simulink model "ContoleLateralApplication_atual"  (R2021a)
settings: Solver=ode23tb  StartTime=0.0  StopTime=TME.Simulation  FixedStep=.001  RelTol=1e-3  EnableMultiTasking=on
StartFcn:
  | %tic
StopFcn:
  | %toc
model workspace (MAT data in the model file):
  A_mu = 10
  B_reff = 8.386
  Cz = 7766.25
  DCT_Param : object (value not decoded)
  DLCXref = [0 6 7 14 33.5 34 42 50 60]
  DLCYref = [0 0 -4.5 -4 -3.75 1.5 0.5 0 0]
  D_reff = 0.25826
  Downshift_Speeds = [9.5625 12.9375 16.3125 19.6875 23.0625 26.4375 29.8125 33.1875 36.5625 39.9375 43.3125 46.6875 ... (28 elements, 4x7)]
  EngRevLim = 7000
  Pedal_Positions = [0.1 0.4 0.5 0.9]
  SUS : object (value not decoded)
  Upshift_Speeds = [12.9375 16.3125 19.6875 33 26.4375 29.8125 33.1875 52.5 39.9375 43.3125 46.6875 77.25 ... (28 elements, 4x7)]
  VEH : object (value not decoded)
  V_o = 16.7
  V_xlow = 1
  WH : object (value not decoded)
  a = 1.4
  alpha_max = 1.5
  alpha_min = -1.5
  b = 1.8
  c_zo = 209651
  epsilon = 0.1
  h = 0.134
  path : object (value not decoded)
  pio = 220000
  q_Fcx = 0
  q_Fz2 = 15.4
  q_Fzy = 0
  q_reo = 0.9974
  q_sx1 = -0.007764
  q_sx10 = 0.2824
  q_sx11 = 5.349
  q_sx12 = 0
  q_sx13 = 0
  q_sx14 = 0
  q_sx2 = 1.1915
  q_sx3 = 0.013948
  q_sx4 = 4.912
  q_sx5 = 1.02
  q_sx6 = 22.83
  q_sx7 = 0.7104
  q_sx8 = -0.023393
  q_sx9 = 0.6581
  q_sy1 = 0.00702
  q_sy2 = 0
  q_sy3 = 0.001515
  q_sy4 = 8.514e-05
  q_sy5 = 0
  q_sy6 = 0
  q_sy7 = 0.9008
  q_sy8 = -0.4089
  q_v1 = 0.0007742
  q_v2 = 0.04667
  r_Bx1 = 12.531
  r_Bx2 = 9.532
  r_Bx3 = 0
  r_By1 = 10.615
  r_By2 = 7.705
  r_By3 = 3.433e-06
  r_By4 = 0
  r_Cx1 = 1.019
  r_Cy1 = 1.0585
  r_Ex1 = -0.4487
  r_Ex2 = -0.4726
  r_Ey1 = 0.3132
  r_Ey2 = 7.63e-06
  r_Hx1 = 0.0002374
  r_Hy1 = 0.011646
  r_Hy2 = 7.63e-06
  r_Vy1 = 0.05654
  r_Vy2 = 7.63e-06
  r_Vy3 = 0
  r_Vy4 = 99.9
  r_Vy5 = 2
  r_Vy6 = 15.814
  r_o = 0.3135
  vehWidth = 2
  w = 1
values from neighbouring files (symbols this model uses):
  C1 = 1.2801    [Data_ControleLateral_atual.m]
  C2 = 23.99    [Data_ControleLateral_atual.m]
  C3 = 0.52    [Data_ControleLateral_atual.m]
symbols that are objects in the model workspace (value not decoded): VEH
undefined symbols (not defined in the file or in its folder): Disabled, EV, GND, MTR, Right, SENSOR, STEER, WHL
libraries: autolibutils x5, vehdynlibscenariocommon x5, autolibshared x5, sim3dlib x4, vehdynlibtirecommon x2, autolibmappedmotor x2, vehdynlibviscommon x2, vehdynlibsteering x1, pid_lib x1, vehdynlibdriver x1, vehdynlibsens x1, sharedtransform x1
(part 5 of 6)

== system ContoleLateralApplication_atual/Veh2Tire ==
  Axle : Inport
  r : Inport  Port=2
  VehVel : Inport  Port=3
  WheelSteer : Inport  Port=4
  Reshape4 : Reshape
  Unary Minus : UnaryMinus
  Wheel to Body Transform : Subsystem
  T : Outport  VectorParamsAs1DForOutWhenUnconnected=off
  xdotAxle : Outport  Port=2  VectorParamsAs1DForOutWhenUnconnected=off
  ydotAxle : Outport  Port=3  VectorParamsAs1DForOutWhenUnconnected=off
  psidot : Outport  Port=4  VectorParamsAs1DForOutWhenUnconnected=off
  zdotAxle : Outport  Port=5  VectorParamsAs1DForOutWhenUnconnected=off
  wires:
  Axle/1 -> Reshape4/1
  Wheel to Body Transform/1(xdotWheel) -> xdotAxle/1  "Vx"
  Wheel to Body Transform/2(ydotWheel) -> ydotAxle/1  "Vy"
  r/1 -> Unary Minus/1
  Reshape4/1 -> T/1
  VehVel/1 -> Wheel to Body Transform/1(VelVeh)
  WheelSteer/1 -> Wheel to Body Transform/2(WheelAngles)
  Wheel to Body Transform/3(zdotWheel) -> zdotAxle/1  "Vz"
  Unary Minus/1 -> psidot/1

== system ContoleLateralApplication_atual/Velocity and Vertical Load ==
  note: 1) Add Subsystem or Model blocks as valid variant choices.
      | 2) You cannot connect blocks at this level. At simulation, connectivity is automatically
      | determined, based on the active variant and port name matching.
  VehFdbk : Inport
  Bicycle : Subsystem  VariantControl=0
  Dual : Subsystem  VariantControl=1
  VehV : Outport  VectorParamsAs1DForOutWhenUnconnected=off
  Fz : Outport  Port=2  PortDimensions=4  VectorParamsAs1DForOutWhenUnconnected=off

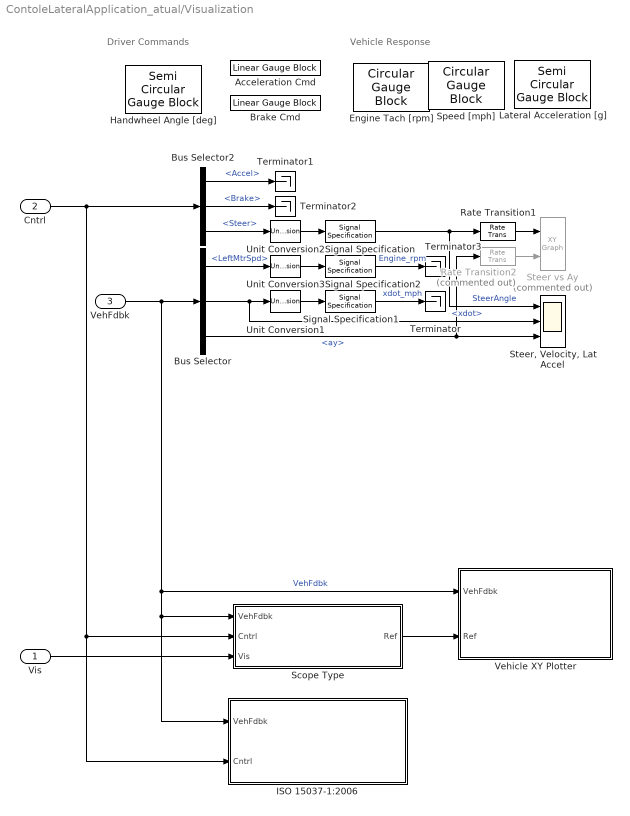
== system ContoleLateralApplication_atual/Visualization ==
  note: Vehicle Response
  note: Driver Commands
  Vis : Inport
  Cntrl : Inport  Port=2
  VehFdbk : Inport  Port=3
  Acceleration Cmd : LinearGaugeBlock  LabelPosition=Hide  ScaleMax=1  TickInterval=0.20000000000000001
  Brake Cmd : LinearGaugeBlock  LabelPosition=Hide  ScaleMax=1  TickInterval=0.20000000000000001
  Bus Selector : BusSelector  OutputSignals=Driveline.LeftMtrSpd,Chassis.xdot,Chassis.ay
  Bus Selector2 : BusSelector  OutputSignals=Accel,Brake,Steer
  Engine Tach [rpm] : CircularGaugeBlock  LabelPosition=Hide  ScaleMax=8000  TickInterval=1000
  Handwheel Angle [deg] : SemiCircularGaugeBlock  LabelPosition=Hide  ScaleMin=-300  ScaleMax=300  TickInterval=60
  ISO 15037-1:2006 : Subsystem  StopFcn=|  Variant=on  VariantControlMode=label  LabelModeActiveChoice=0  mask(ISO 15037-1:2006){Measurement=Disabled}
      | switch get_param(gcb,'Measurement')
      |     case 'Enabled'
      |        p=slproject.getCurrentProject;
      |        projectRoot=p.RootFolder;
      |        SySFolder=fullfile(projectRoot, 'System');
      |        Simulink.sdi.loadView([SySFolder filesep 'ISO15037_1_2006E.mldatx']);
      |        Simulink.sdi.view;
      | end
      mask prompts: Measurement "ISO Measurements"
      mask help: Enables display of ISO 15037-1:2006 standard measurement signals in the Simulation Data Inspector.
      mask init:
      | switch get_param(gcb,'Measurement')
      |     case 'Disabled'
      |         set_param(gcb,'OverrideUsingVariant','0')
      |     case 'Enabled'
      |        set_param(gcb,'OverrideUsingVariant','1')
      |     otherwise
      |        set_param(gcb,'OverrideUsingVariant','0')
      | end
      settings: AttributesFormatString=%<Measurement>
      mask Help: eval('vdynblkshelp(''iso15037'')');
      mask TypeOptions Measurement: Enabled | Disabled
      mask Callback Measurement:
      | switch get_param(gcb,'Measurement')
      |     case 'Disabled'
      |         set_param(gcb,'OverrideUsingVariant','0')
      |     case 'Enabled'
      |        set_param(gcb,'OverrideUsingVariant','1')
      |     otherwise
      |        set_param(gcb,'OverrideUsingVariant','0')
      | end
      mask Display: disp('ISO 15037-1:2006')
  Lateral Acceleration [g] : SemiCircularGaugeBlock  LabelPosition=Hide  ScaleMin=-1  ScaleMax=1  TickInterval=0.5
  Rate Transition1 : RateTransition  Deterministic=off  OutPortSampleTime=.1
  Rate Transition2 : RateTransition  Commented=on  Deterministic=off  OutPortSampleTime=.1
  Scope Type : Subsystem  Variant=on  VariantControlMode=label  VariantControl=Variant1  LabelModeActiveChoice=2
  Signal Specification : SignalSpecification  Unit=deg
  Signal Specification1 : SignalSpecification  Unit=mph
  Signal Specification2 : SignalSpecification  Unit=rpm
  Speed [mph] : CircularGaugeBlock  LabelPosition=Hide  TickInterval=10
  Steer vs Ay : simulink/Sinks/XY Graph  Commented=on  xmin=-300  xmax=300  ymin=-1.5  ymax=1.5  st=.1
  "Steer, Velocity, Lat Accel" : Scope  NumInputPorts=3
  Terminator{,1..3} (4 alike) : Terminator
  Unit Conversion1 : UnitConversion
  Unit Conversion2 : UnitConversion
  Unit Conversion3 : UnitConversion
  Vehicle XY Plotter : Subsystem  Variant=on  VariantControlMode=label  VariantControl=Variant1  LabelModeActiveChoice=1
  wires:
  Signal Specification/1 -> Rate Transition1/1, "Steer, Velocity, Lat Accel"/1  "SteerAngle"
  Bus Selector/3 -> Rate Transition2/1, "Steer, Velocity, Lat Accel"/3  "<ay>"
  Bus Selector/2 -> "Steer, Velocity, Lat Accel"/2, Unit Conversion1/1  "<xdot>"
  Unit Conversion2/1 -> Signal Specification/1
  Unit Conversion1/1 -> Signal Specification1/1
  Signal Specification1/1 -> Terminator/1  "xdot_mph"
  Bus Selector2/3 -> Unit Conversion2/1  "<Steer>"
  Rate Transition1/1 -> Steer vs Ay/1
  Rate Transition2/1 -> Steer vs Ay/2
  Bus Selector2/1 -> Terminator1/1  "<Accel>"
  Bus Selector2/2 -> Terminator2/1  "<Brake>"
  Signal Specification2/1 -> Terminator3/1  "Engine_rpm"
  Unit Conversion3/1 -> Signal Specification2/1
  Bus Selector/1 -> Unit Conversion3/1  "<LeftMtrSpd>"
  VehFdbk/1 -> ISO 15037-1:2006/1(VehFdbk), Scope Type/1("VehFdbk "), Vehicle XY Plotter/1("VehFdbk "), Bus Selector/1  "VehFdbk"
  Cntrl/1 -> ISO 15037-1:2006/2(Cntrl), Scope Type/2(Cntrl), Bus Selector2/1
  Vis/1 -> Scope Type/3("Vis ")
  Scope Type/1(" Ref") -> Vehicle XY Plotter/2("Ref ")

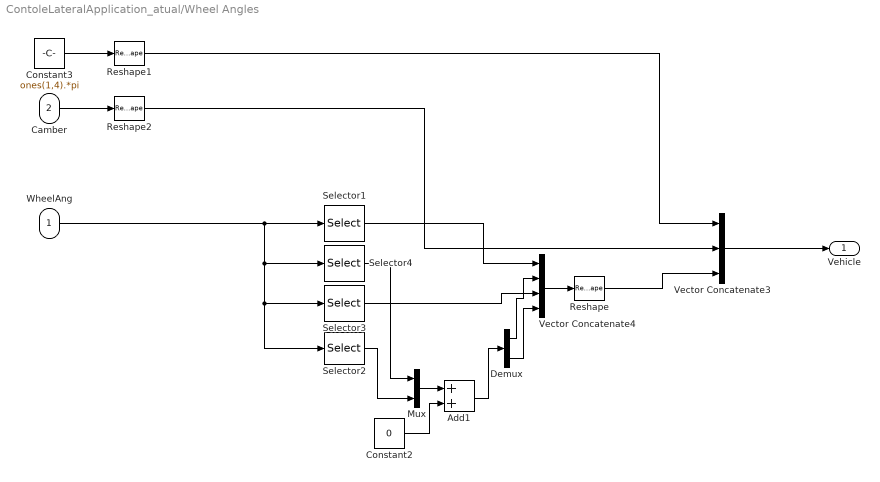
== system ContoleLateralApplication_atual/Wheel Angles ==
  WheelAng : Inport
  Camber : Inport  Port=2
  Add1 : Sum
  Constant2 : Constant  Value=0
  Constant3 : Constant  Value=ones(1,4).*pi
  Demux : Demux  Outputs=2
  Mux : Mux  Inputs=2
  Reshape : Reshape  OutputDimensionality=Row vector (2-D)
  Reshape1 : Reshape  OutputDimensionality=Row vector (2-D)
  Reshape2 : Reshape  OutputDimensionality=Row vector (2-D)
  Selector1 : Selector  InputPortWidth=4  IndexOptions=Index vector (dialog)  Indices=1  OutputSizes=4
  Selector2 : Selector  InputPortWidth=4  IndexOptions=Index vector (dialog)  Indices=4  OutputSizes=4
  Selector3 : Selector  InputPortWidth=4  IndexOptions=Index vector (dialog)  Indices=3  OutputSizes=4
  Selector4 : Selector  InputPortWidth=4  IndexOptions=Index vector (dialog)  Indices=2  OutputSizes=4
  Vector Concatenate3 : Concatenate  NumInputs=3  Mode=Multidimensional array
  Vector Concatenate4 : Concatenate  NumInputs=4
  Vehicle : Outport  VectorParamsAs1DForOutWhenUnconnected=off
  wires:
  Selector4/1 -> Mux/1
  Constant2/1 -> Add1/2
  Add1/1 -> Demux/1
  Selector3/1 -> Vector Concatenate4/3
  Selector1/1 -> Vector Concatenate4/1
  Mux/1 -> Add1/1
  Selector2/1 -> Mux/2
  Demux/1 -> Vector Concatenate4/2
  Demux/2 -> Vector Concatenate4/4
  Vector Concatenate4/1 -> Reshape/1
  Constant3/1 -> Reshape1/1
  Vector Concatenate3/1 -> Vehicle/1
  Reshape/1 -> Vector Concatenate3/3
  Reshape1/1 -> Vector Concatenate3/1
  Reshape2/1 -> Vector Concatenate3/2
  Camber/1 -> Reshape2/1
  WheelAng/1 -> Selector2/1, Selector3/1, Selector4/1, Selector1/1

== system ContoleLateralApplication_atual/Wheel Positions ==
  Info : Inport
  Bus Selector : BusSelector  OutputSignals=InertFrm.FrntAxl.Lft.Disp.Y,InertFrm.FrntAxl.Rght.Disp.Y,InertFrm.RearAxl.Lft.Disp.Y,InertFrm.RearAxl.Rght.Disp.Y
  Bus Selector1 : BusSelector  OutputSignals=InertFrm.FrntAxl.Lft.Disp.X,InertFrm.FrntAxl.Rght.Disp.X,InertFrm.RearAxl.Lft.Disp.X,InertFrm.RearAxl.Rght.Disp.X
  Vector Concatenate1 : Concatenate  NumInputs=4
  Vector Concatenate2 : Concatenate  NumInputs=4
  XWheel : Outport  Unit=m  VectorParamsAs1DForOutWhenUnconnected=off
  YWheel : Outport  Port=2  Unit=m  VectorParamsAs1DForOutWhenUnconnected=off
  wires:
  Bus Selector1/4 -> Vector Concatenate2/4  "<X>"
  Bus Selector/1 -> Vector Concatenate1/1  "<Y>"
  Bus Selector1/3 -> Vector Concatenate2/3  "<X>"
  Bus Selector/4 -> Vector Concatenate1/4  "<Y>"
  Bus Selector1/2 -> Vector Concatenate2/2  "<X>"
  Bus Selector/3 -> Vector Concatenate1/3  "<Y>"
  Bus Selector/2 -> Vector Concatenate1/2  "<Y>"
  Vector Concatenate1/1 -> YWheel/1
  Info/1 -> Bus Selector/1, Bus Selector1/1
  Bus Selector1/1 -> Vector Concatenate2/1  "<X>"
  Vector Concatenate2/1 -> XWheel/1

== system ContoleLateralApplication_atual/Axle Forces/Bicycle ==
  F : Inport
  R : Inport  Port=2
  Sum of Elements : Sum  Inputs=+
  Sum of Elements1 : Sum  Inputs=+
  FrntAxlF : Outport  Unit=N  VectorParamsAs1DForOutWhenUnconnected=off
  RearAxlF : Outport  Port=2  Unit=N  VectorParamsAs1DForOutWhenUnconnected=off
  wires:
  Sum of Elements/1 -> FrntAxlF/1
  Sum of Elements1/1 -> RearAxlF/1
  R/1 -> Sum of Elements1/1
  F/1 -> Sum of Elements/1

== system ContoleLateralApplication_atual/Axle Forces/Dual ==
  F : Inport
  R : Inport  Port=2
  FrntAxlF : Outport  Unit=N  VectorParamsAs1DForOutWhenUnconnected=off
  RearAxlF : Outport  Port=2  Unit=N  VectorParamsAs1DForOutWhenUnconnected=off
  wires:
  R/1 -> RearAxlF/1
  F/1 -> FrntAxlF/1

== system ContoleLateralApplication_atual/Environment/Ground Feedback ==
  note: 1) Add Subsystem or Model blocks as valid variant choices.
      | 2) You cannot connect blocks at this level. At simulation, connectivity is automatically
      | determined, based on the active variant and port name matching.
  Friction : Inport
  3D Engine : Subsystem  VariantControl=1
  Constant : Subsystem  VariantControl=0
  Ground : Outport  VectorParamsAs1DForOutWhenUnconnected=off

== system ContoleLateralApplication_atual/Reference Generator/3D Engine ==
  note: 1) Add Subsystem or Model blocks as valid variant choices.
      | 2) You cannot connect blocks at this level. At simulation, connectivity is automatically
      | determined, based on the active variant and port name matching.
  VehFdbk : Inport
  3D Engine : Subsystem  VariantControl=1
  3D Engine Disabled : Subsystem  VariantControl=0

== system ContoleLateralApplication_atual/Reference Generator/Reference Generator ==
  "VehFdbk " : Inport
  Constant Radius : vehdynlibscenariocommon/Constant Radius  VariantControl=4  t_start=t_start  xdot_r=xdot_r  xdotUnit=mph  R=R  turnDirMask=Right  ay_max=cr_ay_max  ay_stop=off  Parameter6=2
      settings: SourceProductBaseCode=VE
  Double Lane Change : Subsystem  VariantControl=0
  Increasing Steer : Subsystem  VariantControl=1
  Sine with Dwell : Subsystem  VariantControl=3
  Swept Sine : Subsystem  VariantControl=2
  " Vis" : Outport  VectorParamsAs1DForOutWhenUnconnected=off
  " Ref" : Outport  Port=2  VectorParamsAs1DForOutWhenUnconnected=off
  " Fdbk" : Outport  Port=3  VectorParamsAs1DForOutWhenUnconnected=off

== system ContoleLateralApplication_atual/Tires/Fx ==
  In1 : Inport
  In2 : Inport  Port=2
  In3 : Inport  Port=3
  In4 : Inport  Port=4
  Bus Selector{,1..3} (4 alike) : BusSelector  OutputSignals=Fx
  Vector Concatenate : Concatenate  NumInputs=4
  Out1 : Outport  VectorParamsAs1DForOutWhenUnconnected=off
  wires:
  Bus Selector3/1 -> Vector Concatenate/4  "<Fx>"
  Bus Selector2/1 -> Vector Concatenate/3  "<Fx>"
  Bus Selector1/1 -> Vector Concatenate/2  "<Fx>"
  In4/1 -> Bus Selector3/1
  In3/1 -> Bus Selector2/1
  In2/1 -> Bus Selector1/1
  Bus Selector/1 -> Vector Concatenate/1  "<Fx>"
  In1/1 -> Bus Selector/1
  Vector Concatenate/1 -> Out1/1

== system ContoleLateralApplication_atual/Tires/Fz1 ==
  In1 : Inport
  In2 : Inport  Port=2
  In3 : Inport  Port=3
  In4 : Inport  Port=4
  Bus Selector{,1..3} (4 alike) : BusSelector  OutputSignals=Fz
  Vector Concatenate : Concatenate  NumInputs=4
  Out1 : Outport  VectorParamsAs1DForOutWhenUnconnected=off
  wires:
  Vector Concatenate/1 -> Out1/1
  In1/1 -> Bus Selector/1
  Bus Selector/1 -> Vector Concatenate/1  "<Fz>"
  In2/1 -> Bus Selector1/1
  In3/1 -> Bus Selector2/1
  In4/1 -> Bus Selector3/1
  Bus Selector1/1 -> Vector Concatenate/2  "<Fz>"
  Bus Selector2/1 -> Vector Concatenate/3  "<Fz>"
  Bus Selector3/1 -> Vector Concatenate/4  "<Fz>"

== system ContoleLateralApplication_atual/Tires/My ==
  In1 : Inport
  In2 : Inport  Port=2
  In3 : Inport  Port=3
  In4 : Inport  Port=4
  Bus Selector{,1..3} (4 alike) : BusSelector  OutputSignals=My
  Vector Concatenate : Concatenate  NumInputs=4
  Out1 : Outport  PortDimensions=4  VectorParamsAs1DForOutWhenUnconnected=off
  wires:
  Bus Selector3/1 -> Vector Concatenate/4  "<My>"
  Bus Selector2/1 -> Vector Concatenate/3  "<My>"
  Bus Selector1/1 -> Vector Concatenate/2  "<My>"
  In4/1 -> Bus Selector3/1
  In3/1 -> Bus Selector2/1
  In2/1 -> Bus Selector1/1
  Bus Selector/1 -> Vector Concatenate/1  "<My>"
  In1/1 -> Bus Selector/1
  Vector Concatenate/1 -> Out1/1

== system ContoleLateralApplication_atual/Tires/Re ==
  In1 : Inport
  In2 : Inport  Port=2
  In3 : Inport  Port=3
  In4 : Inport  Port=4
  Bus Selector{,1..3} (4 alike) : BusSelector  OutputSignals=Re
  Vector Concatenate : Concatenate  NumInputs=4
  Out1 : Outport  PortDimensions=4  VectorParamsAs1DForOutWhenUnconnected=off
  wires:
  Vector Concatenate/1 -> Out1/1
  In1/1 -> Bus Selector/1
  Bus Selector/1 -> Vector Concatenate/1  "<Re>"
  In2/1 -> Bus Selector1/1
  In3/1 -> Bus Selector2/1
  In4/1 -> Bus Selector3/1
  Bus Selector1/1 -> Vector Concatenate/2  "<Re>"
  Bus Selector2/1 -> Vector Concatenate/3  "<Re>"
  Bus Selector3/1 -> Vector Concatenate/4  "<Re>"

== system ContoleLateralApplication_atual/Tires/alpha ==
  In1 : Inport
  In2 : Inport  Port=2
  In3 : Inport  Port=3
  In4 : Inport  Port=4
  Vector Concatenate : Concatenate  NumInputs=4
  Out1 : Outport  PortDimensions=4  VectorParamsAs1DForOutWhenUnconnected=off
  wires:
  Vector Concatenate/1 -> Out1/1
  In1/1 -> Vector Concatenate/1
  In2/1 -> Vector Concatenate/2
  In3/1 -> Vector Concatenate/3
  In4/1 -> Vector Concatenate/4

== system ContoleLateralApplication_atual/Tires/kappa ==
  In1 : Inport
  In2 : Inport  Port=2
  In3 : Inport  Port=3
  In4 : Inport  Port=4
  Bus Selector{,1..3} (4 alike) : BusSelector  OutputSignals=Kappa
  Vector Concatenate : Concatenate  NumInputs=4
  Out1 : Outport  PortDimensions=4  VectorParamsAs1DForOutWhenUnconnected=off
  wires:
  Bus Selector3/1 -> Vector Concatenate/4  "<Kappa>"
  Bus Selector2/1 -> Vector Concatenate/3  "<Kappa>"
  Bus Selector1/1 -> Vector Concatenate/2  "<Kappa>"
  In4/1 -> Bus Selector3/1
  In3/1 -> Bus Selector2/1
  In2/1 -> Bus Selector1/1
  Bus Selector/1 -> Vector Concatenate/1  "<Kappa>"
  In1/1 -> Bus Selector/1
  Vector Concatenate/1 -> Out1/1

== system ContoleLateralApplication_atual/Tires/omega ==
  In1 : Inport
  In2 : Inport  Port=2
  In3 : Inport  Port=3
  In4 : Inport  Port=4
  Bus Selector{1..4} (4 alike) : BusSelector  OutputSignals=Omega
  Vector Concatenate : Concatenate  NumInputs=4
  Out1 : Outport  VectorParamsAs1DForOutWhenUnconnected=off
  wires:
  In1/1 -> Bus Selector4/1
  Bus Selector4/1 -> Vector Concatenate/1  "<Omega>"
  In2/1 -> Bus Selector2/1
  In3/1 -> Bus Selector1/1
  In4/1 -> Bus Selector3/1
  Bus Selector2/1 -> Vector Concatenate/2  "<Omega>"
  Vector Concatenate/1 -> Out1/1
  Bus Selector3/1 -> Vector Concatenate/4  "<Omega>"
  Bus Selector1/1 -> Vector Concatenate/3  "<Omega>"

== system ContoleLateralApplication_atual/Tires/z ==
  In1 : Inport
  In2 : Inport  Port=2
  In3 : Inport  Port=3
  In4 : Inport  Port=4
  Bus Selector{,1..3} (4 alike) : BusSelector  OutputSignals=z
  Vector Concatenate : Concatenate  NumInputs=4
  Out1 : Outport  PortDimensions=4  VectorParamsAs1DForOutWhenUnconnected=off
  wires:
  Bus Selector3/1 -> Vector Concatenate/4  "<z>"
  Bus Selector2/1 -> Vector Concatenate/3  "<z>"
  Bus Selector1/1 -> Vector Concatenate/2  "<z>"
  In4/1 -> Bus Selector3/1
  In3/1 -> Bus Selector2/1
  In2/1 -> Bus Selector1/1
  Bus Selector/1 -> Vector Concatenate/1  "<z>"
  In1/1 -> Bus Selector/1
  Vector Concatenate/1 -> Out1/1

== system ContoleLateralApplication_atual/Tires/zdot ==
  In1 : Inport
  In2 : Inport  Port=2
  In3 : Inport  Port=3
  In4 : Inport  Port=4
  Bus Selector{,1..3} (4 alike) : BusSelector  OutputSignals=zdot
  Vector Concatenate : Concatenate  NumInputs=4
  Out1 : Outport  PortDimensions=4  VectorParamsAs1DForOutWhenUnconnected=off
  wires:
  Vector Concatenate/1 -> Out1/1
  In1/1 -> Bus Selector/1
  Bus Selector/1 -> Vector Concatenate/1  "<zdot>"
  In2/1 -> Bus Selector1/1
  In3/1 -> Bus Selector2/1
  In4/1 -> Bus Selector3/1
  Bus Selector1/1 -> Vector Concatenate/2  "<zdot>"
  Bus Selector2/1 -> Vector Concatenate/3  "<zdot>"
  Bus Selector3/1 -> Vector Concatenate/4  "<zdot>"

== system ContoleLateralApplication_atual/Veh2Tire/Wheel to Body Transform ==
  VelVeh : Inport  Partition=on  PartitionDimension=2  PartitionWidth=1  PartitionOffset=0
  WheelAngles : Inport  Port=2  Partition=on  PartitionDimension=2  PartitionWidth=1  PartitionOffset=0
  Demux1 : Demux  Outputs=3
  Divide1 : Product  Inputs=**  Multiplication=Matrix(*)
  For Each : ForEach  DisableCoverage=on
  Rotation Angles to Direction Cosine Matrix : sharedtransform/Rotation Angles to Direction Cosine Matrix  rotationOrder=ZYX  aMode=2
      settings: SourceProductBaseCode=AE,PW,DR,MT,UV,VE
  Selector : Selector  InputPortWidth=3  IndexOptions=Index vector (dialog)  Indices=[3 2 1]  OutputSizes=1
  xdotWheel : Outport  ConcatenationDimension=1  VectorParamsAs1DForOutWhenUnconnected=off
  ydotWheel : Outport  Port=2  ConcatenationDimension=1  VectorParamsAs1DForOutWhenUnconnected=off
  zdotWheel : Outport  Port=3  ConcatenationDimension=1  VectorParamsAs1DForOutWhenUnconnected=off
  wires:
  Divide1/1 -> Demux1/1
  Demux1/1 -> xdotWheel/1
  Demux1/2 -> ydotWheel/1
  Demux1/3 -> zdotWheel/1
  Rotation Angles to Direction Cosine Matrix/1 -> Divide1/1
  VelVeh/1 -> Divide1/2
  WheelAngles/1 -> Selector/1
  Selector/1 -> Rotation Angles to Direction Cosine Matrix/1

== system ContoleLateralApplication_atual/Velocity and Vertical Load/Bicycle ==
  VehFdbk : Inport
  Bicycle Fz : Subsystem
  Bicycle V : Subsystem
  VehV : Outport  VectorParamsAs1DForOutWhenUnconnected=off
  Fz : Outport  Port=2  VectorParamsAs1DForOutWhenUnconnected=off
  wires:
  Bicycle V/1(Out1) -> VehV/1
  Bicycle Fz/1(Out1) -> Fz/1
  VehFdbk/1 -> Bicycle Fz/1(In1), Bicycle V/1(In1)

== system ContoleLateralApplication_atual/Velocity and Vertical Load/Dual ==
  VehFdbk : Inport
  Dual Fz : Subsystem
  Dual V : Subsystem
  VehV : Outport  VectorParamsAs1DForOutWhenUnconnected=off
  Fz : Outport  Port=2  VectorParamsAs1DForOutWhenUnconnected=off
  wires:
  Dual V/1(Out1) -> VehV/1
  VehFdbk/1 -> Dual Fz/1(In1), Dual V/1(In1)
  Dual Fz/1(Out1) -> Fz/1

== system ContoleLateralApplication_atual/Visualization/ISO 15037-1:2006 ==
  VehFdbk : Inport
  Cntrl : Inport  Port=2
  Disabled : Subsystem  VariantControl=0
  Enabled : Subsystem  VariantControl=1

== system ContoleLateralApplication_atual/Visualization/Scope Type ==
  "VehFdbk " : Inport
  Cntrl : Inport  Port=2
  "Vis " : Inport  Port=3
  DLC : Subsystem  VariantControl=1
  None : Subsystem  VariantControl=0
  XYZ : Subsystem  VariantControl=2
  " Ref" : Outport  VectorParamsAs1DForOutWhenUnconnected=off

== system ContoleLateralApplication_atual/Visualization/Vehicle XY Plotter ==
  "VehFdbk " : Inport
  "Ref " : Inport  Port=2
  XY View : Subsystem  VariantControl=0
  XY View Ref : Subsystem  VariantControl=1

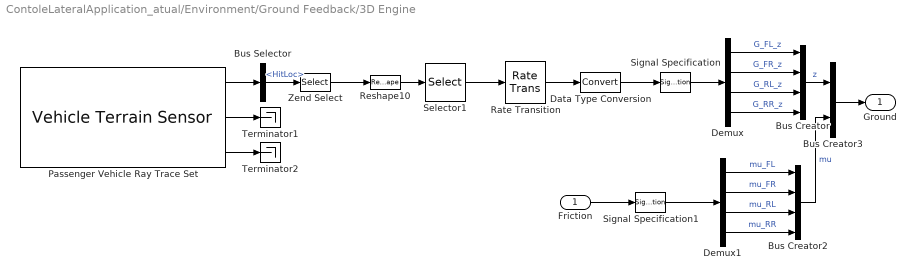
== system ContoleLateralApplication_atual/Environment/Ground Feedback/3D Engine ==
  Friction : Inport
  Bus Creator : BusCreator  Inputs=4
  Bus Creator2 : BusCreator  Inputs=4
  Bus Creator3 : BusCreator  Inputs=2
  Bus Selector : BusSelector  OutputSignals=HitLoc
  Data Type Conversion : DataTypeConversion
  Demux : Demux
  Demux1 : Demux
  Passenger Vehicle Ray Trace Set : sim3dlib/Vehicle Terrain Sensor  ActorTag=SimulinkVehicle1  VehExtEn=Constant  TireRadiiExt=Constant  VehCntrLngthVal=0  TireRadiiVal=0  VehRayLngth=10  LfRayLngth=20  RfRayLngth=20  LrRayLngth=20  RrRayLngth=20  VehRayOffset=0  LfRayOffset=-1  RfRayOffset=-1  LrRayOffset=-1  RrRayOffset=-1  VehEn=on  LfEn=on  RfEn=on  LrEn=on  RrEn=on  DbgEn=off  Ts=.03  aMode=aMode
      settings: SourceProductBaseCode=DR,UV,VE
  Rate Transition : RateTransition
  Reshape10 : Reshape  OutputDimensionality=Row vector (2-D)
  Selector1 : Selector  InputPortWidth=5  IndexOptions=Index vector (dialog)  Indices=[2:5]  OutputSizes=1
  Signal Specification : SignalSpecification  Unit=m
  Signal Specification1 : SignalSpecification  Unit=1
  Terminator1 : Terminator
  Terminator2 : Terminator
  Zend Select : Selector  NumberOfDimensions=2  InputPortWidth=3  IndexOptions=Select all,Index vector (dialog)  Indices=[1 3],3  OutputSizes=1,1
  Ground : Outport  VectorParamsAs1DForOutWhenUnconnected=off
  wires:
  Selector1/1 -> Rate Transition/1
  Zend Select/1 -> Reshape10/1
  Bus Selector/1 -> Zend Select/1  "<HitLoc>"
  Passenger Vehicle Ray Trace Set/2 -> Terminator1/1
  Passenger Vehicle Ray Trace Set/3 -> Terminator2/1
  Reshape10/1 -> Selector1/1
  Passenger Vehicle Ray Trace Set/1 -> Bus Selector/1
  Rate Transition/1 -> Data Type Conversion/1
  Demux/2 -> Bus Creator/2  "G_FR_z"
  Demux/1 -> Bus Creator/1  "G_FL_z"
  Demux/4 -> Bus Creator/4  "G_RR_z"
  Demux/3 -> Bus Creator/3  "G_RL_z"
  Signal Specification/1 -> Demux/1
  Signal Specification1/1 -> Demux1/1
  Demux1/1 -> Bus Creator2/1  "mu_FL"
  Bus Creator/1 -> Bus Creator3/1  "z"
  Demux1/3 -> Bus Creator2/3  "mu_RL"
  Demux1/4 -> Bus Creator2/4  "mu_RR"
  Demux1/2 -> Bus Creator2/2  "mu_FR"
  Bus Creator2/1 -> Bus Creator3/2  "mu"
  Bus Creator3/1 -> Ground/1
  Friction/1 -> Signal Specification1/1
  Data Type Conversion/1 -> Signal Specification/1

== system ContoleLateralApplication_atual/Environment/Ground Feedback/Constant ==
  Friction : Inport
  Bus Creator : BusCreator  Inputs=4
  Bus Creator2 : BusCreator  Inputs=4
  Bus Creator3 : BusCreator  Inputs=2
  Constant1 : Constant  Value=zeros(4,1)
  Demux : Demux
  Demux1 : Demux
  Signal Specification : SignalSpecification  Unit=m
  Signal Specification1 : SignalSpecification  Unit=1
  Ground : Outport  VectorParamsAs1DForOutWhenUnconnected=off
  wires:
  Constant1/1 -> Signal Specification/1
  Signal Specification/1 -> Demux/1
  Demux/4 -> Bus Creator/4  "G_RR_z"
  Demux/1 -> Bus Creator/1  "G_FL_z"
  Demux/3 -> Bus Creator/3  "G_RL_z"
  Demux/2 -> Bus Creator/2  "G_FR_z"
  Bus Creator/1 -> Bus Creator3/1  "z"
  Demux1/3 -> Bus Creator2/3  "mu_RL"
  Demux1/4 -> Bus Creator2/4  "mu_RR"
  Demux1/1 -> Bus Creator2/1  "mu_FL"
  Demux1/2 -> Bus Creator2/2  "mu_FR"
  Bus Creator2/1 -> Bus Creator3/2  "mu"
  Friction/1 -> Signal Specification1/1
  Signal Specification1/1 -> Demux1/1
  Bus Creator3/1 -> Ground/1

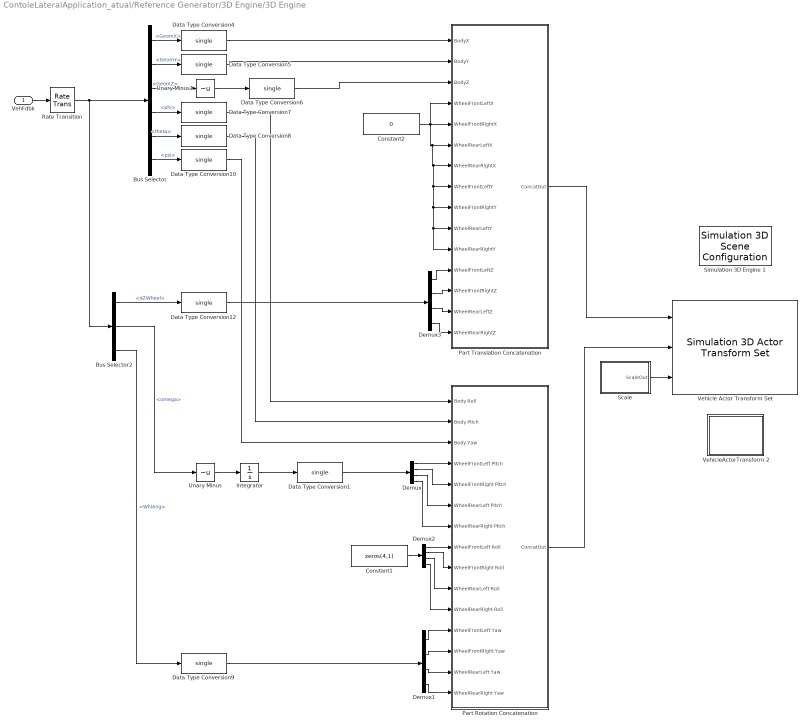
== system ContoleLateralApplication_atual/Reference Generator/3D Engine/3D Engine ==
  VehFdbk : Inport
  Bus Selector : BusSelector  OutputSignals=Body.GeomX,Body.GeomY,Body.GeomZ,Body.phi,Body.theta,Body.psi
  Bus Selector2 : BusSelector  OutputSignals=Wheels.dZWheel,Wheels.omega,Driveline.WhlAng
  Constant1 : Constant  Value=zeros(4,1)  OutDataTypeStr=single
  Constant2 : Constant  Value=0  OutDataTypeStr=single
  Data Type Conversion{1,4..10,12} (9 alike) : DataTypeConversion  OutDataTypeStr=single
  Demux{,1..3} (4 alike) : Demux
  Integrator : Integrator  WrapState=on  WrappedStateUpperValue=2*pi  WrappedStateLowerValue=0  ZeroCross=off
  Part Rotation Concatenation : Subsystem
  Part Translation Concatenation : Subsystem
  Rate Transition : RateTransition  OutPortSampleTime=dt3D
  Scale : Subsystem
  Simulation 3D Engine 1 : sim3dlib/Simulation 3D Scene Configuration  Priority=1  ProjectFormat=Default Scenes  SceneDesc=Straight road  ProjectName=C:\Program Files\MATLAB\R2021a\toolbox\shared\sim3d_projects\automotive_project\UE4\WindowsNoEditor\VehicleSimulation.exe  ScenePath=/Game/Maps/HwStrght  vehTagList={'Scene Origin'}  vehTag=Scene Origin  OpVisEn=off  Ts=dt3D  EnableWindow=on  EnableWeather=off  SunAltitude=40.0  SunAzimuth=90  clouds=10  wind=1  fog=0  rain=0  sensorTag=MainCamera1  sensorId=1  sensorName=MainCamera1  mountLoc=Origin  offsetFlag=off  tmountOffset=[0, 0, 0]  rmountOffset=[0, 0, 0]  HorizontalResolution=1280  VerticalResolution=720  HorizontalFOV=60  mountPoint=[0 0 0]  mountOrientation=[0 0 0]  aMode=aMode  ID=1
      settings: AttributesFormatString=Priority: %<Priority>  SourceProductBaseCode=DR,UV,VE
  Unary Minus : UnaryMinus
  Unary Minus1 : UnaryMinus
  Vehicle Actor Transform Set : sim3dlib/Simulation 3D Actor Transform Set  ActorTag=SimulinkVehicle1  NumberOfParts=5  CustNumOfParts=3  Translation=[X_o Y_o -Z_o; 0 0 0; 0 0 0; 0 0 0; 0 0 0]  Rotation=[phi_o theta_o psi_o; 0 0 0; 0 0 0; 0 0 0; 0 0 0]  Scale=[1 1 1; 1 1 1; 1 1 1; 1 1 1; 1 1 1]  Ts=dt3D  aMode=1
      settings: SourceProductBaseCode=DR,UV,VE
  VehicleActorTransform 2 : Subsystem  mask{depth=-5}
      mask prompts: depth "Initital Z position, depth (m):"
  wires:
  Unary Minus1/1 -> Data Type Conversion6/1
  Unary Minus/1 -> Integrator/1
  Bus Selector2/1 -> Data Type Conversion12/1  "<dZWheel>"
  Rate Transition/1 -> Bus Selector/1, Bus Selector2/1
  Scale/1(ScaleOut) -> Vehicle Actor Transform Set/3
  Demux/4 -> Part Rotation Concatenation/7(WheelRearRight Ptich)
  Demux/3 -> Part Rotation Concatenation/6(WheelRearLeft Pitch)
  Demux/2 -> Part Rotation Concatenation/5(WheelFrontRight Pitch)
  Demux/1 -> Part Rotation Concatenation/4(WheelFrontLeft Pitch)
  Constant1/1 -> Demux2/1
  Bus Selector/4 -> Data Type Conversion7/1  "<phi>"
  Part Rotation Concatenation/1(ConcatOut) -> Vehicle Actor Transform Set/2
  Part Translation Concatenation/1(ConcatOut) -> Vehicle Actor Transform Set/1
  Data Type Conversion12/1 -> Demux3/1
  Demux3/4 -> Part Translation Concatenation/15(WheelRearRightZ)
  Demux3/3 -> Part Translation Concatenation/14(WheelRearLeftZ)
  Demux3/1 -> Part Translation Concatenation/12(WheelFrontLeftZ)
  Demux3/2 -> Part Translation Concatenation/13(WheelFrontRightZ)
  VehFdbk/1 -> Rate Transition/1
  Data Type Conversion6/1 -> Part Translation Concatenation/3(BodyZ)
  Demux1/4 -> Part Rotation Concatenation/15(WheelRearRight Yaw)
  Demux1/3 -> Part Rotation Concatenation/14(WheelRearLeft Yaw)
  Demux2/1 -> Part Rotation Concatenation/8(WheelFrontLeft Roll)
  Demux2/2 -> Part Rotation Concatenation/9(WheelFrontRight Roll)
  Demux2/3 -> Part Rotation Concatenation/10(WheelRearLeft Roll)
  Demux2/4 -> Part Rotation Concatenation/11(WheelRearRight Roll)
  Bus Selector2/3 -> Data Type Conversion9/1  "<WhlAng>"
  Bus Selector2/2 -> Unary Minus/1  "<omega>"
  Data Type Conversion9/1 -> Demux1/1
  Demux1/1 -> Part Rotation Concatenation/12(WheelFrontLeft Yaw)
  Demux1/2 -> Part Rotation Concatenation/13(WheelFrontRight Yaw)
  Integrator/1 -> Data Type Conversion1/1
  Data Type Conversion1/1 -> Demux/1
  Data Type Conversion8/1 -> Part Rotation Concatenation/2(Body Ptich)
  Data Type Conversion5/1 -> Part Translation Concatenation/2(BodyY)
  Data Type Conversion10/1 -> Part Rotation Concatenation/3(Body Yaw)
  Constant2/1 -> Part Translation Concatenation/5(WheelFrontRightX), Part Translation Concatenation/6(WheelRearLeftX), Part Translation Concatenation/7(WheelRearRightX), Part Translation Concatenation/8(WheelFrontLeftY), Part Translation Concatenation/9(WheelFrontRightY), Part Translation Concatenation/10(WheelRearLeftY), Part Translation Concatenation/11(WheelRearRightY), Part Translation Concatenation/4(WheelFrontLeftX)
  Data Type Conversion4/1 -> Part Translation Concatenation/1(BodyX)
  Data Type Conversion7/1 -> Part Rotation Concatenation/1(Body Roll)
  Bus Selector/1 -> Data Type Conversion4/1  "<GeomX>"
  Bus Selector/2 -> Data Type Conversion5/1  "<GeomY>"
  Bus Selector/3 -> Unary Minus1/1  "<GeomZ>"
  Bus Selector/6 -> Data Type Conversion10/1  "<psi>"
  Bus Selector/5 -> Data Type Conversion8/1  "<theta>"

== system ContoleLateralApplication_atual/Reference Generator/3D Engine/3D Engine Disabled ==
  VehFdbk : Inport
  Terminator : Terminator
  wires:
  VehFdbk/1 -> Terminator/1

== system ContoleLateralApplication_atual/Reference Generator/Reference Generator/Double Lane Change ==
  "VehFdbk " : Inport
  Double Lane Change : vehdynlibscenariocommon/Lane Change Reference Generator  VariantControl=Variant1  ssMode=Initialize from model  ssVar=dlcSS35mph  t_start=t_start  XGate=XGate  xdot_r=xdot_r  xdotUnit=mph  xStart=xStart  vehW=vehW  latoff=0  lattoff=lattoff  centerSwitch=on  xSimStop=off  latRefbp=latRefbp  latRef=latRef  X_o=0  Y_o=3.125  psi_o=0  ssTol=1  ssMaxTime=30  ssWSName=dlcSS35mph  aMode=2
      settings: SourceProductBaseCode=VE
  " Vis" : Outport  VectorParamsAs1DForOutWhenUnconnected=off
  " Ref" : Outport  Port=2  VectorParamsAs1DForOutWhenUnconnected=off
  " Fdbk" : Outport  Port=3  VectorParamsAs1DForOutWhenUnconnected=off
  wires:
  Double Lane Change/2 -> " Ref"/1
  Double Lane Change/1 -> " Vis"/1
  "VehFdbk "/1 -> Double Lane Change/1, " Fdbk"/1

== system ContoleLateralApplication_atual/Reference Generator/Reference Generator/Increasing Steer ==
  "VehFdbk " : Inport
  Bus Creator : BusCreator  Inputs=3
  Ground : Ground
  Ground1 : Ground
  Ground2 : Ground
  Increasing Steer : vehdynlibscenariocommon/Slowly Increasing Steer  VariantControl=1  ssMode=Initialize from model  ssVar=is50mph  t_start=t_start  xdot_r=xdot_r  xdotUnit=mph  omega_hw=omega_hw  theta_max=theta_max  t_stop=t_stop  ay_max=ay_max  ay_stop=on  X_o=0  Y_o=0  psi_o=0  ssTol=1  ssMaxTime=30  ssWSName=is50mph  aMode=2
      settings: SourceProductBaseCode=VE
  " Vis" : Outport  VectorParamsAs1DForOutWhenUnconnected=off
  " Ref" : Outport  Port=2  VectorParamsAs1DForOutWhenUnconnected=off
  " Fdbk" : Outport  Port=3  VectorParamsAs1DForOutWhenUnconnected=off
  wires:
  Ground/1 -> Bus Creator/1  "XRef"
  Ground1/1 -> Bus Creator/2  "YRef"
  Ground2/1 -> Bus Creator/3  "ZRef"
  Increasing Steer/1 -> " Ref"/1  "LtrlRef"
  Bus Creator/1 -> " Vis"/1
  "VehFdbk "/1 -> Increasing Steer/1, " Fdbk"/1

== system ContoleLateralApplication_atual/Reference Generator/Reference Generator/Sine with Dwell ==
  "VehFdbk " : Inport
  Bus Creator : BusCreator  Inputs=3
  Ground : Ground
  Ground1 : Ground
  Ground2 : Ground
  Sine With Dwell : vehdynlibscenariocommon/Sine With Dwell  VariantControl=3  ssMode=Initialize from model  ssVar=swd50mph  t_start=t_start  xdot_r=xdot_r  xdotUnit=mph  steerF=steerF  steerA=steerA  tdwell=tdwell  steerDir=off  X_o=0  Y_o=0  psi_o=0  ssTol=1  ssMaxTime=30  ssWSName=swd50mph  aMode=2
      settings: SourceProductBaseCode=VE
  " Vis" : Outport  VectorParamsAs1DForOutWhenUnconnected=off
  " Ref" : Outport  Port=2  VectorParamsAs1DForOutWhenUnconnected=off
  " Fdbk" : Outport  Port=3  VectorParamsAs1DForOutWhenUnconnected=off
  wires:
  Ground/1 -> Bus Creator/1  "XRef"
  Ground1/1 -> Bus Creator/2  "YRef"
  Ground2/1 -> Bus Creator/3  "ZRef"
  Bus Creator/1 -> " Vis"/1
  "VehFdbk "/1 -> Sine With Dwell/1, " Fdbk"/1
  Sine With Dwell/1 -> " Ref"/1

== system ContoleLateralApplication_atual/Reference Generator/Reference Generator/Swept Sine ==
  "VehFdbk " : Inport
  Bus Creator : BusCreator  Inputs=3
  Ground : Ground
  Ground1 : Ground
  Ground2 : Ground
  Swept Sine : vehdynlibscenariocommon/Swept Sine Reference Generator  VariantControl=2  ssMode=Initialize from model  ssVar=ss30mph  t_start=t_start  xdot_r=xdot_r  xdotUnit=mph  theta_hw=theta_hw  theta_hw_final=theta_hw_final  t_sweep=t_sweep  X_o=0  Y_o=0  psi_o=0  ssTol=1  ssMaxTime=30  ssWSName=ss30mph  aMode=2
      settings: SourceProductBaseCode=VE
  " Vis" : Outport  VectorParamsAs1DForOutWhenUnconnected=off
  " Ref" : Outport  Port=2  VectorParamsAs1DForOutWhenUnconnected=off
  " Fdbk" : Outport  Port=3  VectorParamsAs1DForOutWhenUnconnected=off
  wires:
  Ground/1 -> Bus Creator/1  "XRef"
  Ground1/1 -> Bus Creator/2  "YRef"
  Ground2/1 -> Bus Creator/3  "ZRef"
  Bus Creator/1 -> " Vis"/1
  Swept Sine/1 -> " Ref"/1
  "VehFdbk "/1 -> Swept Sine/1, " Fdbk"/1

== system ContoleLateralApplication_atual/Velocity and Vertical Load/Bicycle/Bicycle Fz ==
  In1 : Inport
  Bus Selector6 : BusSelector  OutputSignals=BdyFrm.Forces.Tires.FrntTire.Fz,BdyFrm.Forces.Tires.RearTire.Fz
  Cont LPF : autolibutils/Cont LPF  wc=20*2*pi  aMode=2
      settings: SourceProductBaseCode=PW,DR,MT,UV,VE
  Mux5 : Mux
  Saturation : Saturate  UpperLimit=20e3  LowerLimit=1000  ZeroCross=off
  Out1 : Outport  VectorParamsAs1DForOutWhenUnconnected=off
  wires:
  Cont LPF/1 -> Out1/1
  Saturation/1 -> Cont LPF/1
  Bus Selector6/2 -> Mux5/4, Mux5/3  "<Fz>"
  In1/1 -> Bus Selector6/1
  Bus Selector6/1 -> Mux5/2, Mux5/1  "<Fz>"
  Mux5/1 -> Saturation/1

== system ContoleLateralApplication_atual/Velocity and Vertical Load/Bicycle/Bicycle V ==
  In1 : Inport
  Bus Selector : BusSelector  OutputSignals=BdyFrm.FrntAxl.Vel.xdot,BdyFrm.FrntAxl.Vel.ydot,BdyFrm.FrntAxl.Vel.zdot  OutputAsBus=on
  Bus Selector3 : BusSelector  OutputSignals=BdyFrm.RearAxl.Vel.xdot,BdyFrm.RearAxl.Vel.ydot,BdyFrm.RearAxl.Vel.zdot  OutputAsBus=on
  Bus to Vector1 : BusToVector
  Bus to Vector3 : BusToVector
  Vector Concatenate1 : Concatenate  NumInputs=4  Mode=Multidimensional array  ConcatenateDimension=2
  Out1 : Outport  VectorParamsAs1DForOutWhenUnconnected=off
  wires:
  Bus Selector3/1 -> Bus to Vector3/1
  Bus to Vector1/1 -> Vector Concatenate1/2, Vector Concatenate1/1
  In1/1 -> Bus Selector3/1, Bus Selector/1
  Bus Selector/1 -> Bus to Vector1/1
  Bus to Vector3/1 -> Vector Concatenate1/4, Vector Concatenate1/3
  Vector Concatenate1/1 -> Out1/1

== system ContoleLateralApplication_atual/Velocity and Vertical Load/Dual/Dual Fz ==
  In1 : Inport
  Bus Selector6 : BusSelector  OutputSignals=BdyFrm.Forces.Tires.FrntTires.Lft.Fz,BdyFrm.Forces.Tires.FrntTires.Rght.Fz,BdyFrm.Forces.Tires.RearTires.Lft.Fz,BdyFrm.Forces.Tires.RearTires.Rght.Fz
  Cont LPF : autolibutils/Cont LPF  wc=20*2*pi  aMode=2
      settings: SourceProductBaseCode=PW,DR,MT,UV,VE
  Saturation : Saturate  UpperLimit=20e3  LowerLimit=1000  ZeroCross=off
  Vector Concatenate : Concatenate  NumInputs=4
  Out1 : Outport  VectorParamsAs1DForOutWhenUnconnected=off
  wires:
  In1/1 -> Bus Selector6/1
  Saturation/1 -> Cont LPF/1
  Cont LPF/1 -> Out1/1
  Vector Concatenate/1 -> Saturation/1
  Bus Selector6/2 -> Vector Concatenate/2  "<Fz>"
  Bus Selector6/1 -> Vector Concatenate/1  "<Fz>"
  Bus Selector6/3 -> Vector Concatenate/3  "<Fz>"
  Bus Selector6/4 -> Vector Concatenate/4  "<Fz>"

== system ContoleLateralApplication_atual/Velocity and Vertical Load/Dual/Dual V ==
  In1 : Inport
  Bus Selector1 : BusSelector  OutputSignals=BdyFrm.FrntAxl.Lft.Vel.xdot,BdyFrm.FrntAxl.Lft.Vel.ydot,BdyFrm.FrntAxl.Lft.Vel.zdot  OutputAsBus=on
  Bus Selector2 : BusSelector  OutputSignals=BdyFrm.FrntAxl.Rght.Vel.xdot,BdyFrm.FrntAxl.Rght.Vel.ydot,BdyFrm.FrntAxl.Rght.Vel.zdot  OutputAsBus=on
  Bus Selector4 : BusSelector  OutputSignals=BdyFrm.RearAxl.Lft.Vel.xdot,BdyFrm.RearAxl.Lft.Vel.ydot,BdyFrm.RearAxl.Lft.Vel.zdot  OutputAsBus=on
  Bus Selector5 : BusSelector  OutputSignals=BdyFrm.RearAxl.Rght.Vel.xdot,BdyFrm.RearAxl.Rght.Vel.ydot,BdyFrm.RearAxl.Rght.Vel.zdot  OutputAsBus=on
  Bus to Vector{5..8} (4 alike) : BusToVector
  Vector Concatenate2 : Concatenate  NumInputs=4  Mode=Multidimensional array  ConcatenateDimension=2
  Out1 : Outport  VectorParamsAs1DForOutWhenUnconnected=off
  wires:
  Bus to Vector6/1 -> Vector Concatenate2/2
  Bus Selector2/1 -> Bus to Vector6/1
  Bus to Vector8/1 -> Vector Concatenate2/4
  Bus Selector4/1 -> Bus to Vector7/1
  Bus to Vector5/1 -> Vector Concatenate2/1
  Bus Selector1/1 -> Bus to Vector5/1
  In1/1 -> Bus Selector1/1, Bus Selector2/1, Bus Selector4/1, Bus Selector5/1
  Bus Selector5/1 -> Bus to Vector8/1
  Bus to Vector7/1 -> Vector Concatenate2/3
  Vector Concatenate2/1 -> Out1/1

== system ContoleLateralApplication_atual/Visualization/ISO 15037-1:2006/Disabled ==
  VehFdbk : Inport
  Cntrl : Inport  Port=2
  Terminator : Terminator
  Terminator1 : Terminator
  wires:
  Cntrl/1 -> Terminator/1
  VehFdbk/1 -> Terminator1/1

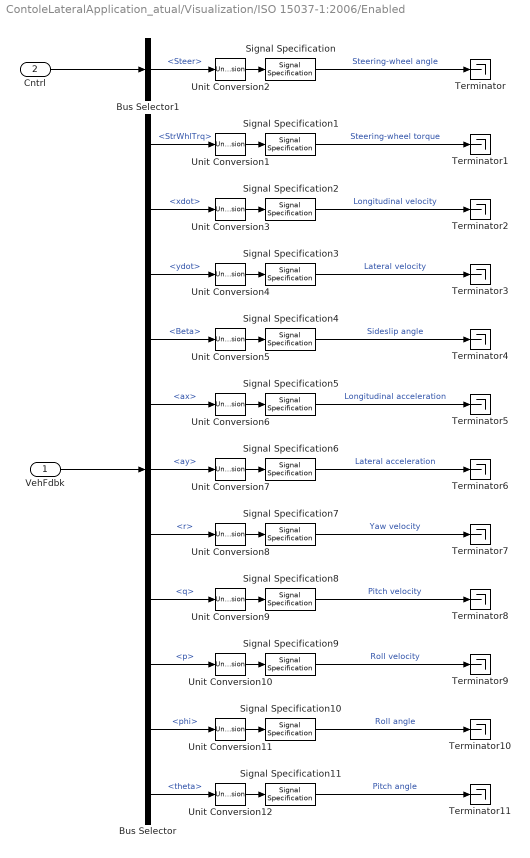
== system ContoleLateralApplication_atual/Visualization/ISO 15037-1:2006/Enabled ==
  VehFdbk : Inport
  Cntrl : Inport  Port=2
  Bus Selector : BusSelector  OutputSignals=Steering.StrWhlTrq,Chassis.xdot,Chassis.ydot,Chassis.Beta,Chassis.ax,Chassis.ay,Chassis.r,Chassis.q,Chassis.p,Chassis.phi,Chassis.theta
  Bus Selector1 : BusSelector  OutputSignals=Steer
  Signal Specification{,4,10..11} (4 alike) : SignalSpecification  Unit=deg
  Signal Specification1 : SignalSpecification  Unit=N*m
  Signal Specification2 : SignalSpecification  Unit=km/h
  Signal Specification3 : SignalSpecification  Unit=m/s
  Signal Specification5 : SignalSpecification  Unit=m/s^2
  Signal Specification6 : SignalSpecification  Unit=m/s^2
  Signal Specification7 : SignalSpecification  Unit=deg/s
  Signal Specification8 : SignalSpecification  Unit=deg/s
  Signal Specification9 : SignalSpecification  Unit=deg/s
  Terminator{,1..11} (12 alike) : Terminator
  Unit Conversion{1..12} (12 alike) : UnitConversion
  wires:
  Bus Selector/11 -> Unit Conversion12/1  "<theta>"
  Signal Specification11/1 -> Terminator11/1  "Pitch angle"
  Unit Conversion12/1 -> Signal Specification11/1
  Bus Selector/10 -> Unit Conversion11/1  "<phi>"
  Unit Conversion11/1 -> Signal Specification10/1
  Signal Specification10/1 -> Terminator10/1  "Roll angle"
  Bus Selector/9 -> Unit Conversion10/1  "<p>"
  Signal Specification9/1 -> Terminator9/1  "Roll velocity"
  Unit Conversion10/1 -> Signal Specification9/1
  Bus Selector/8 -> Unit Conversion9/1  "<q>"
  Unit Conversion9/1 -> Signal Specification8/1
  Signal Specification8/1 -> Terminator8/1  "Pitch velocity"
  Bus Selector/7 -> Unit Conversion8/1  "<r>"
  Signal Specification7/1 -> Terminator7/1  "Yaw velocity"
  Unit Conversion8/1 -> Signal Specification7/1
  Bus Selector/6 -> Unit Conversion7/1  "<ay>"
  Unit Conversion7/1 -> Signal Specification6/1
  Signal Specification6/1 -> Terminator6/1  "Lateral acceleration"
  Bus Selector/5 -> Unit Conversion6/1  "<ax>"
  Signal Specification5/1 -> Terminator5/1  "Longitudinal acceleration"
  Unit Conversion6/1 -> Signal Specification5/1
  Bus Selector/4 -> Unit Conversion5/1  "<Beta>"
  Unit Conversion5/1 -> Signal Specification4/1
  Signal Specification4/1 -> Terminator4/1  "Sideslip angle"
  Bus Selector/3 -> Unit Conversion4/1  "<ydot>"
  Signal Specification3/1 -> Terminator3/1  "Lateral velocity"
  Unit Conversion4/1 -> Signal Specification3/1
  Bus Selector/2 -> Unit Conversion3/1  "<xdot>"
  Unit Conversion3/1 -> Signal Specification2/1
  Signal Specification2/1 -> Terminator2/1  "Longitudinal velocity"
  Signal Specification1/1 -> Terminator1/1  "Steering-wheel torque"
  Unit Conversion1/1 -> Signal Specification1/1
  Bus Selector/1 -> Unit Conversion1/1  "<StrWhlTrq>"
  Signal Specification/1 -> Terminator/1  "Steering-wheel angle"
  Unit Conversion2/1 -> Signal Specification/1
  Bus Selector1/1 -> Unit Conversion2/1  "<Steer>"
  Cntrl/1 -> Bus Selector1/1
  VehFdbk/1 -> Bus Selector/1

== system ContoleLateralApplication_atual/Visualization/Scope Type/DLC ==
  VehFdbk : Inport
  Vis : Inport  Port=2
  Bus Creator : BusCreator  Inputs=3
  Bus Selector3 : BusSelector  OutputSignals=Chassis.Y,Chassis.X,Chassis.Z
  Bus Selector4 : BusSelector  OutputSignals=UB,LB,LtrlRef
  Lane Change : Scope
  Mux1 : Mux
  Signal Copy : SignalConversion  OverrideOpt=off
  Signal Copy1 : SignalConversion  OverrideOpt=off
  Signal Copy2 : SignalConversion  OverrideOpt=off
  Ref : Outport  VectorParamsAs1DForOutWhenUnconnected=off
  wires:
  Bus Selector4/1 -> Mux1/1  "<UB>"
  Bus Selector3/1 -> Mux1/4  "<Y>"
  VehFdbk/1 -> Bus Selector3/1
  Mux1/1 -> Lane Change/1
  Vis/1 -> Bus Selector4/1
  Bus Selector4/3 -> Signal Copy/1, Mux1/3  "<LtrlRef>"
  Bus Selector4/2 -> Mux1/2  "<LB>"
  Bus Selector3/2 -> Signal Copy1/1  "<X>"
  Bus Creator/1 -> Ref/1
  Bus Selector3/3 -> Signal Copy2/1  "<Z>"
  Signal Copy/1 -> Bus Creator/2  "YRef"
  Signal Copy1/1 -> Bus Creator/1  "XRef"
  Signal Copy2/1 -> Bus Creator/3  "ZRef"

== system ContoleLateralApplication_atual/Visualization/Scope Type/None ==
  VehFdbk : Inport
  Vis : Inport  Port=2
  Cntrl : Inport  Port=3
  Bus Selector1 : BusSelector  OutputSignals=Steer
  Bus Selector9 : BusSelector  OutputSignals=Chassis.r
  Signal Specification3 : SignalSpecification  Unit=deg/s
  Unit Conversion4 : UnitConversion
  Yaw Rate and Steer : Scope  NumInputPorts=2
  Ref : Outport  VectorParamsAs1DForOutWhenUnconnected=off
  wires:
  Bus Selector9/1 -> Unit Conversion4/1  "<r>"
  Signal Specification3/1 -> Yaw Rate and Steer/1
  Unit Conversion4/1 -> Signal Specification3/1
  VehFdbk/1 -> Bus Selector9/1  "VehFdbk"
  Bus Selector1/1 -> Yaw Rate and Steer/2  "<Steer>"
  Vis/1 -> Ref/1
  Cntrl/1 -> Bus Selector1/1

== system ContoleLateralApplication_atual/Visualization/Scope Type/XYZ ==
  VehFdbk : Inport
  Vis : Inport  Port=2
  Terminator : Terminator
  Ref : Outport  VectorParamsAs1DForOutWhenUnconnected=off
  wires:
  Vis/1 -> Ref/1
  VehFdbk/1 -> Terminator/1

== system ContoleLateralApplication_atual/Visualization/Vehicle XY Plotter/XY View ==
  VehFdbk : Inport
  Bus Selector1 : BusSelector  OutputSignals=Chassis.phi,Chassis.theta,Chassis.psi  OutputAsBus=on
  Bus Selector5 : BusSelector  OutputSignals=Driveline.WhlAng  OutputAsBus=on
  Bus Selector6 : BusSelector  OutputSignals=Chassis.GeomX,Chassis.GeomY,Chassis.GeomZ  OutputAsBus=on
  Bus Selector7 : BusSelector  OutputSignals=Chassis.GeomXdot,Chassis.GeomYdot,Chassis.GeomZdot  OutputAsBus=on
  Bus to Vector : BusToVector
  Bus to Vector1 : BusToVector
  Bus to Vector2 : BusToVector
  Vehicle XY Plotter : Subsystem  mask(Vehicle XY Plotter){a=VEH.FrontAxlePositionfromCG, b=VEH.RearAxlePositionfromCG, w=VEH.TrackWidth, figBorder=10, bufferSize=1024, extRef=off, pltDT=.1}
      mask prompts: a "Distance to front axle from CG, a [m]:"; b "Distance to rear axle from CG, b [m]:"; w "Track width, w [m]:"; figBorder "Distance to figure borders, figBorder [m]:"; bufferSize "Path buffer sampe size, bufferSize []:"; extRef "Plot path reference, extRef"; pltDT "Plot update rate, pltDT [s]:"
      mask help:
      | This block will display a MATLAB figure which indicates the vehicle path, current position and heading velocity.
      | An optional path reference is also provided.
      mask init:
      | if autoblkschecksimstopped(gcb)
      |     PortName = 'RefXYZ';
      |     InportOption  = {'built-in/Ground', [PortName, ' Ground'];...
      |         'built-in/Inport',PortName };
      |     if ~strcmp(get_param(gcb,'extRef'),'on')
      |         NewBlkHdl = autoblksreplaceblock(gcb, InportOption, 1);
      |         set_param(NewBlkHdl, 'ShowName', 'off');
      |     else
      |         autoblksreplaceblock(gcb, InportOption, 2);
      |     end
      | end
      mask TypeOptions a: Vehicle XY Plotter/a
      mask TypeOptions b: Vehicle XY Plotter/b
      mask TypeOptions w: Vehicle XY Plotter/w
      mask TypeOptions figBorder: Vehicle XY Plotter/figBorder
      mask TypeOptions bufferSize: Vehicle XY Plotter/bufferSize
  wires:
  Bus to Vector2/1 -> Vehicle XY Plotter/2(InertAng)
  Bus to Vector/1 -> Vehicle XY Plotter/1(InertXYZ)
  Bus Selector5/1 -> Vehicle XY Plotter/4(delta)
  Bus Selector1/1 -> Bus to Vector2/1
  Bus Selector6/1 -> Bus to Vector/1
  Bus Selector7/1 -> Bus to Vector1/1
  VehFdbk/1 -> Bus Selector6/1, Bus Selector1/1, Bus Selector7/1, Bus Selector5/1
  Bus to Vector1/1 -> Vehicle XY Plotter/3(InertXdotYdotZdot)

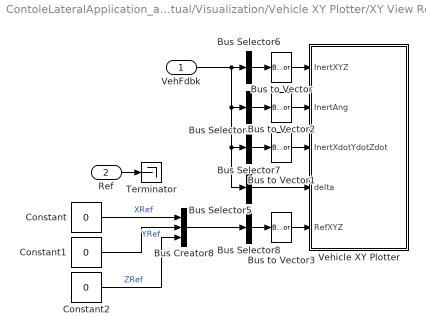
== system ContoleLateralApplication_atual/Visualization/Vehicle XY Plotter/XY View Ref ==
  VehFdbk : Inport
  Ref : Inport  Port=2
  Bus Creator8 : BusCreator  Inputs=3
  Bus Selector1 : BusSelector  OutputSignals=Chassis.phi,Chassis.theta,Chassis.psi  OutputAsBus=on
  Bus Selector5 : BusSelector  OutputSignals=Driveline.WhlAng  OutputAsBus=on
  Bus Selector6 : BusSelector  OutputSignals=Chassis.GeomX,Chassis.GeomY,Chassis.GeomZ  OutputAsBus=on
  Bus Selector7 : BusSelector  OutputSignals=Chassis.GeomXdot,Chassis.GeomYdot,Chassis.GeomZdot  OutputAsBus=on
  Bus Selector8 : BusSelector  OutputSignals=XRef,YRef,ZRef  OutputAsBus=on
  Bus to Vector{,1..3} (4 alike) : BusToVector
  Constant : Constant  Value=0
  Constant1 : Constant  Value=0
  Constant2 : Constant  Value=0
  Terminator : Terminator
  Vehicle XY Plotter : Subsystem  mask(Vehicle XY Plotter){a=EV.FrontAxlePositionfromCG, b=EV.RearAxlePositionfromCG, w=EV.TrackWidth(1), figBorder=10, bufferSize=1024, extRef=on, pltDT=.1}
      mask prompts: a "Distance to front axle from CG, a [m]:"; b "Distance to rear axle from CG, b [m]:"; w "Track width, w [m]:"; figBorder "Distance to figure borders, figBorder [m]:"; bufferSize "Path buffer sampe size, bufferSize []:"; extRef "Plot path reference, extRef"; pltDT "Plot update rate, pltDT [s]:"
      mask help:
      | This block will display a MATLAB figure which indicates the vehicle path, current position and heading velocity.
      | An optional path reference is also provided.
      mask init: same as ContoleLateralApplication_atual/Visualization/Vehicle XY Plotter/XY View/Vehicle XY Plotter
      mask TypeOptions a: Vehicle XY Plotter/a
      mask TypeOptions b: Vehicle XY Plotter/b
      mask TypeOptions w: Vehicle XY Plotter/w
      mask TypeOptions figBorder: Vehicle XY Plotter/figBorder
      mask TypeOptions bufferSize: Vehicle XY Plotter/bufferSize
  wires:
  Bus Selector8/1 -> Bus to Vector3/1
  Bus to Vector1/1 -> Vehicle XY Plotter/3(InertXdotYdotZdot)
  VehFdbk/1 -> Bus Selector5/1, Bus Selector7/1, Bus Selector1/1, Bus Selector6/1
  Bus Selector7/1 -> Bus to Vector1/1
  Bus Selector6/1 -> Bus to Vector/1
  Bus Selector1/1 -> Bus to Vector2/1
  Bus Selector5/1 -> Vehicle XY Plotter/4(delta)
  Bus to Vector/1 -> Vehicle XY Plotter/1(InertXYZ)
  Bus to Vector2/1 -> Vehicle XY Plotter/2(InertAng)
  Bus to Vector3/1 -> Vehicle XY Plotter/5(RefXYZ)
  Constant/1 -> Bus Creator8/1  "XRef"
  Constant1/1 -> Bus Creator8/2  "YRef"
  Constant2/1 -> Bus Creator8/3  "ZRef"
  Bus Creator8/1 -> Bus Selector8/1
  Ref/1 -> Terminator/1
